simulink model "SerialComm"  (R2022a)
settings: Solver=FixedStepAuto  StartTime=0.0  StopTime=10.0  FixedStep=1e-3  RelTol=1e-3  EnableMultiTasking=on
undefined symbols (not defined in the file): A0, A1, D0, D1, D10, D11, D12, D13, D2, D3, D4, D5, D6, D7, D8, D9, PTA0, PTA1, PTA2, PTB2, PTB23, PTB3, PTB9, PTC16, PTC17, PTC2, PTC3, PTC4, PTD0, PTD1, PTD2, PTD3
libraries: frdmk64flib x19, svdutilitieslib x4, dspstat3 x1
settings Model: ExtModeTrigDuration=5  Creator=haotianxue  LastModifiedBy=1wanj
settings OptimizationCC: EnhancedBackFolding=on  PassReuseOutputArgsAs=Individual arguments  ZeroExternalMemoryAtStartup=off  ZeroInternalMemoryAtStartup=off  MaxStackSize=64  OptimizeBlockOrder=speed  DifferentSizesBufferReuse=on  OptimizationCustomize=off  EfficientTunableParamExpr=on
settings DebuggingCC: ParameterTunabilityLossMsg=error  UnconnectedInputMsg=warning  UnconnectedOutputMsg=warning  UnconnectedLineMsg=warning
settings HardwareCC: ProdBitPerPointer=32  ProdBitPerSizeT=32  ProdBitPerPtrDiffT=32  ProdLargestAtomicInteger=Long  ProdLargestAtomicFloat=Double  ProdWordSize=32  ProdHWDeviceType=ARM Compatible->ARM Cortex
settings SFSimCC: MATLABDynamicMemAlloc=off
settings RTWCC: SystemTargetFile=ert.tlc  HardwareBoard=NXP FRDM-K64F  TLCOptions="-aInlineSetEventsForThisBaseRateFcn=TLC_FALSE -aSuppressMultiTaskScheduler=TLC_FALSE  -aRateBasedStepFcn=0"  TemplateMakefile=ert_default_tmf  Toolchain=GNU Tools for ARM Embedded Processors  DLArmComputeVersion=19.05
settings CodeAppCC: ForceParamTrailComments=on  IgnoreCustomStorageClasses=off  OperatorAnnotations=on  SimulinkDataObjDesc=on  SFDataObjDesc=on  InsertBlockDesc=on
settings ERTTargetCC: ExtModeTransport=4  ExtModeMexFile=sendToCommService

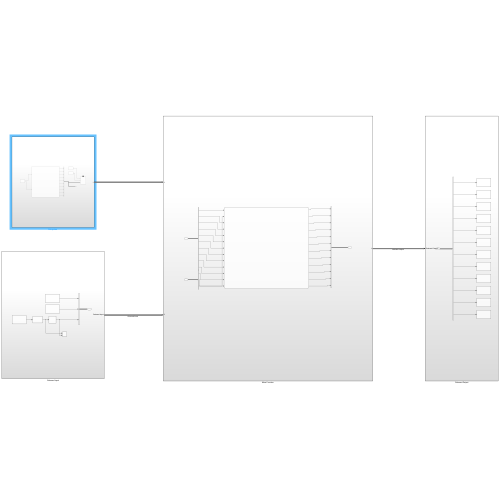
[thumbnail: Simulink's stored preview of the top-level diagram]
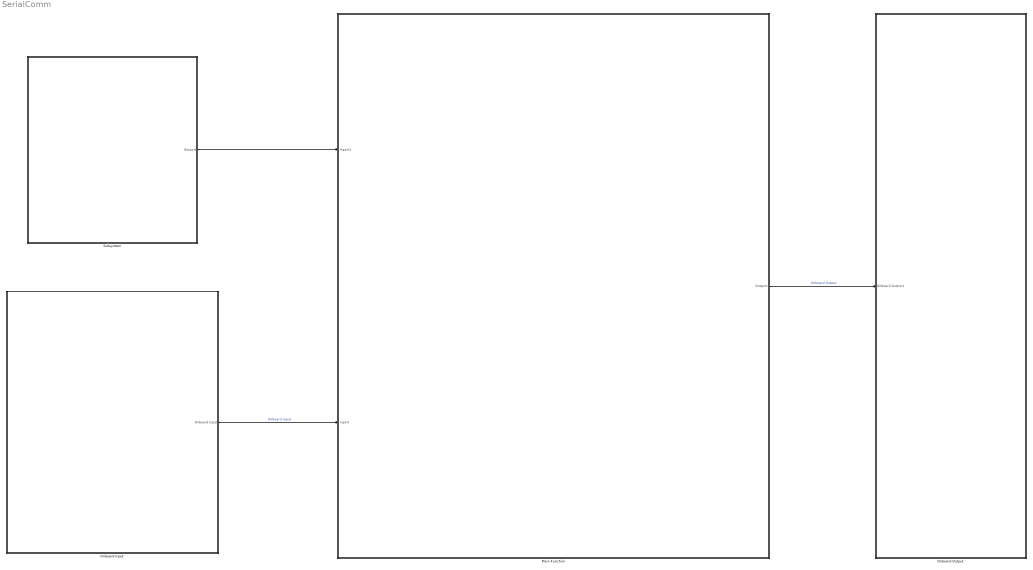
== system SerialComm ==
  Main Function : Subsystem
  Onboard Input : Subsystem
  Onboard Output : Subsystem
  Subsystem : Subsystem
  wires:
  Onboard Input/1(Onboard Input) -> Main Function/2(Inport)  "Onboard Input"
  Main Function/1(Outport) -> Onboard Output/1(Onboard Outport)  "Onboard Output"
  Subsystem/1(Outport) -> Main Function/1(Inport1)

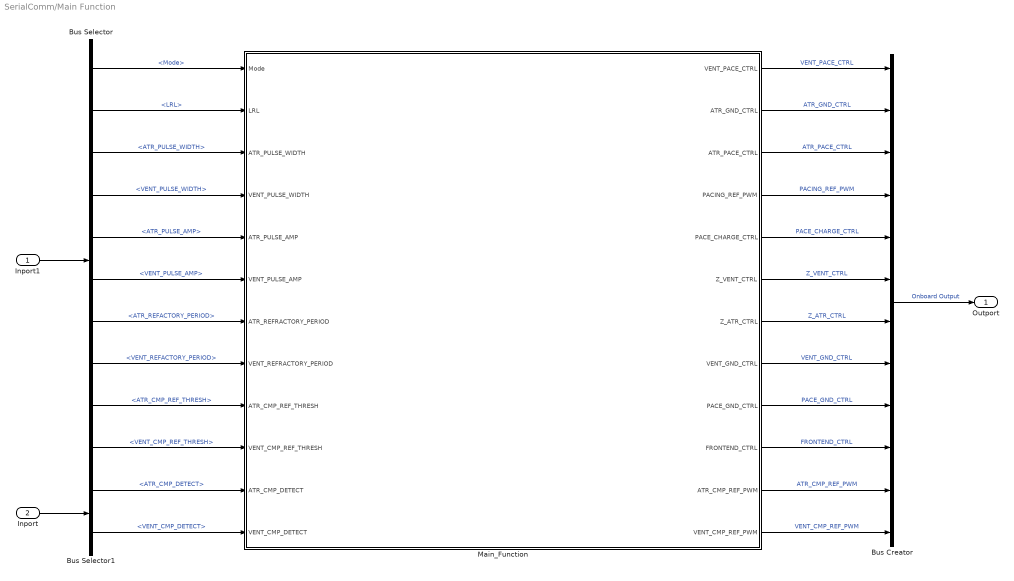
== system SerialComm/Main Function ==
  Inport1 : Inport
  Inport : Inport  Port=2
  Bus Creator : BusCreator  Inputs=12
  Bus Selector : BusSelector  OutputSignals=Mode,LRL,ATR_PULSE_WIDTH,VENT_PULSE_WIDTH,ATR_PULSE_AMP,VENT_PULSE_AMP,ATR_REFACTORY_PERIOD,VENT_REFACTORY_PERIOD,ATR_CMP_REF_THRESH,VENT_CMP_REF_THRESH
  Bus Selector1 : BusSelector  OutputSignals=ATR_CMP_DETECT,VENT_CMP_DETECT
  Main_Function : Stateflow chart  TreatAsAtomicUnit=on
  Outport : Outport
  wires:
  Main_Function/8(VENT_GND_CTRL) -> Bus Creator/8  "VENT_GND_CTRL"
  Main_Function/1(VENT_PACE_CTRL) -> Bus Creator/1  "VENT_PACE_CTRL"
  Bus Selector/1 -> Main_Function/1(Mode)  "<Mode>"
  Bus Selector/3 -> Main_Function/3(ATR_PULSE_WIDTH)  "<ATR_PULSE_WIDTH>"
  Bus Selector/4 -> Main_Function/4(VENT_PULSE_WIDTH)  "<VENT_PULSE_WIDTH>"
  Bus Selector1/1 -> Main_Function/11(ATR_CMP_DETECT)  "<ATR_CMP_DETECT>"
  Main_Function/9(PACE_GND_CTRL) -> Bus Creator/9  "PACE_GND_CTRL"
  Main_Function/7(Z_ATR_CTRL) -> Bus Creator/7  "Z_ATR_CTRL"
  Main_Function/6(Z_VENT_CTRL) -> Bus Creator/6  "Z_VENT_CTRL"
  Main_Function/5(PACE_CHARGE_CTRL) -> Bus Creator/5  "PACE_CHARGE_CTRL"
  Main_Function/4(PACING_REF_PWM) -> Bus Creator/4  "PACING_REF_PWM"
  Main_Function/3(ATR_PACE_CTRL) -> Bus Creator/3  "ATR_PACE_CTRL"
  Main_Function/2(ATR_GND_CTRL) -> Bus Creator/2  "ATR_GND_CTRL"
  Inport1/1 -> Bus Selector/1
  Inport/1 -> Bus Selector1/1
  Bus Creator/1 -> Outport/1  "Onboard Output"
  Bus Selector/5 -> Main_Function/5(ATR_PULSE_AMP)  "<ATR_PULSE_AMP>"
  Bus Selector/6 -> Main_Function/6(VENT_PULSE_AMP)  "<VENT_PULSE_AMP>"
  Main_Function/10(FRONTEND_CTRL) -> Bus Creator/10  "FRONTEND_CTRL"
  Main_Function/11(ATR_CMP_REF_PWM) -> Bus Creator/11  "ATR_CMP_REF_PWM"
  Main_Function/12(VENT_CMP_REF_PWM) -> Bus Creator/12  "VENT_CMP_REF_PWM"
  Bus Selector/9 -> Main_Function/9(ATR_CMP_REF_THRESH)  "<ATR_CMP_REF_THRESH>"
  Bus Selector/10 -> Main_Function/10(VENT_CMP_REF_THRESH)  "<VENT_CMP_REF_THRESH>"
  Bus Selector/2 -> Main_Function/2(LRL)  "<LRL>"
  Bus Selector1/2 -> Main_Function/12(VENT_CMP_DETECT)  "<VENT_CMP_DETECT>"
  Bus Selector/7 -> Main_Function/7(ATR_REFRACTORY_PERIOD)  "<ATR_REFACTORY_PERIOD>"
  Bus Selector/8 -> Main_Function/8(VENT_REFRACTORY_PERIOD)  "<VENT_REFACTORY_PERIOD>"

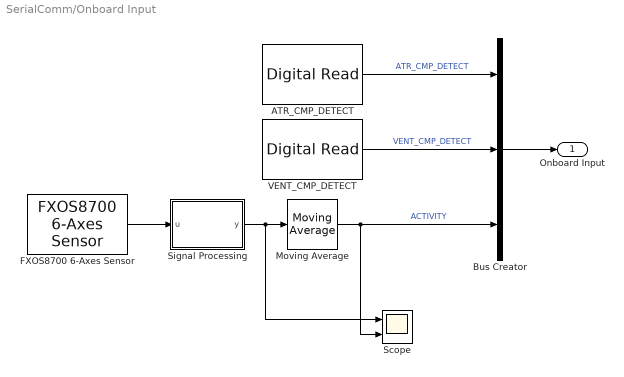
== system SerialComm/Onboard Input ==
  ATR_CMP_DETECT : frdmk64flib/Digital Read  Whichpin=PTC16 (D0)  SampleTime=-1
  Bus Creator : BusCreator  Inputs=3
  FXOS8700 6-Axes Sensor : frdmk64flib/FXOS8700 6-Axes Sensor  Activesensor=Accelerometer only  ODR=800Hz  HybridODR=400Hz  Accelfullrange=-4g to +4g  SampleTime=-1
  Moving Average : dspstat3/Moving Average  Method=Sliding window  ForgettingFactorPort=off  SpecifyWindowLength=on  WindowLength=30  ForgettingFactor=0.9  SimulateUsing=Code generation
  Scope : Scope  NumInputPorts=2
  Signal Processing : MATLAB Function  TreatAsAtomicUnit=on
  VENT_CMP_DETECT : frdmk64flib/Digital Read  Whichpin=PTC17 (D1)  SampleTime=-1
  Onboard Input : Outport
  wires:
  VENT_CMP_DETECT/1 -> Bus Creator/2  "VENT_CMP_DETECT"
  ATR_CMP_DETECT/1 -> Bus Creator/1  "ATR_CMP_DETECT"
  Bus Creator/1 -> Onboard Input/1
  FXOS8700 6-Axes Sensor/1 -> Signal Processing/1(u)
  Signal Processing/1(y) -> Scope/1, Moving Average/1
  Moving Average/1 -> Scope/2, Bus Creator/3  "ACTIVITY"

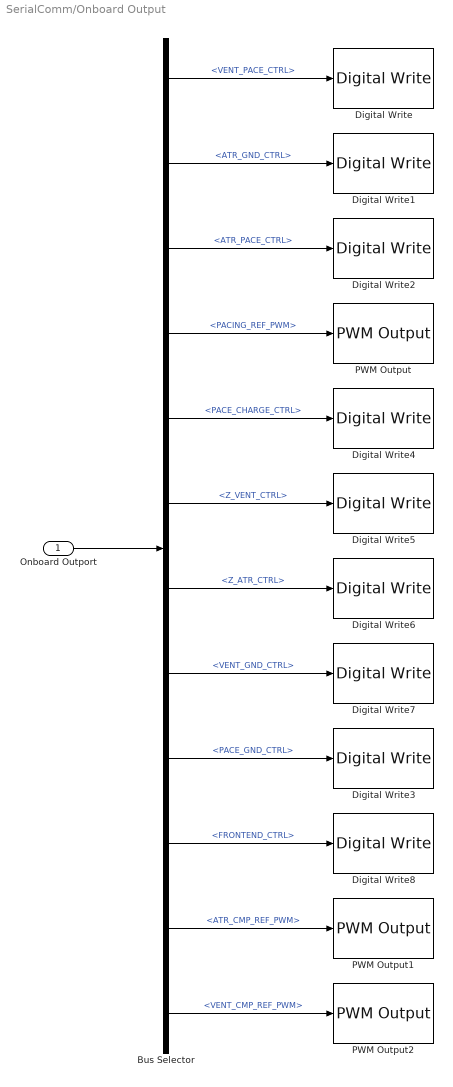
== system SerialComm/Onboard Output ==
  Onboard Outport : Inport
  Bus Selector : BusSelector  OutputSignals=VENT_PACE_CTRL,ATR_GND_CTRL,ATR_PACE_CTRL,PACING_REF_PWM,PACE_CHARGE_CTRL,Z_VENT_CTRL,Z_ATR_CTRL,VENT_GND_CTRL,PACE_GND_CTRL,FRONTEND_CTRL,ATR_CMP_REF_PWM,VENT_CMP_REF_PWM
  Digital Write : frdmk64flib/Digital Write  Whichpin=PTC4 (D9)
  Digital Write1 : frdmk64flib/Digital Write  Whichpin=PTD2 (D11)
  Digital Write2 : frdmk64flib/Digital Write  Whichpin=PTA0 (D8)
  Digital Write3 : frdmk64flib/Digital Write  Whichpin=PTD0 (D10)
  Digital Write4 : frdmk64flib/Digital Write  Whichpin=PTB9 (D2)
  Digital Write5 : frdmk64flib/Digital Write  Whichpin=PTC3 (D7)
  Digital Write6 : frdmk64flib/Digital Write  Whichpin=PTB23 (D4)
  Digital Write7 : frdmk64flib/Digital Write  Whichpin=PTD3 (D12)
  Digital Write8 : frdmk64flib/Digital Write  Whichpin=PTD1 (D13)
  PWM Output : frdmk64flib/PWM Output  Whichpin=PTA2 (D5)  InitialFrequency=2000  InitialDutyCycle=50
  PWM Output1 : frdmk64flib/PWM Output  Whichpin=PTC2 (D6)  InitialFrequency=2000  InitialDutyCycle=50
  PWM Output2 : frdmk64flib/PWM Output  Whichpin=PTA1 (D3)  InitialFrequency=2000  InitialDutyCycle=50
  wires:
  Onboard Outport/1 -> Bus Selector/1
  Bus Selector/1 -> Digital Write/1  "<VENT_PACE_CTRL>"
  Bus Selector/2 -> Digital Write1/1  "<ATR_GND_CTRL>"
  Bus Selector/3 -> Digital Write2/1  "<ATR_PACE_CTRL>"
  Bus Selector/4 -> PWM Output/1  "<PACING_REF_PWM>"
  Bus Selector/5 -> Digital Write4/1  "<PACE_CHARGE_CTRL>"
  Bus Selector/6 -> Digital Write5/1  "<Z_VENT_CTRL>"
  Bus Selector/7 -> Digital Write6/1  "<Z_ATR_CTRL>"
  Bus Selector/8 -> Digital Write7/1  "<VENT_GND_CTRL>"
  Bus Selector/9 -> Digital Write3/1  "<PACE_GND_CTRL>"
  Bus Selector/10 -> Digital Write8/1  "<FRONTEND_CTRL>"
  Bus Selector/11 -> PWM Output1/1  "<ATR_CMP_REF_PWM>"
  Bus Selector/12 -> PWM Output2/1  "<VENT_CMP_REF_PWM>"

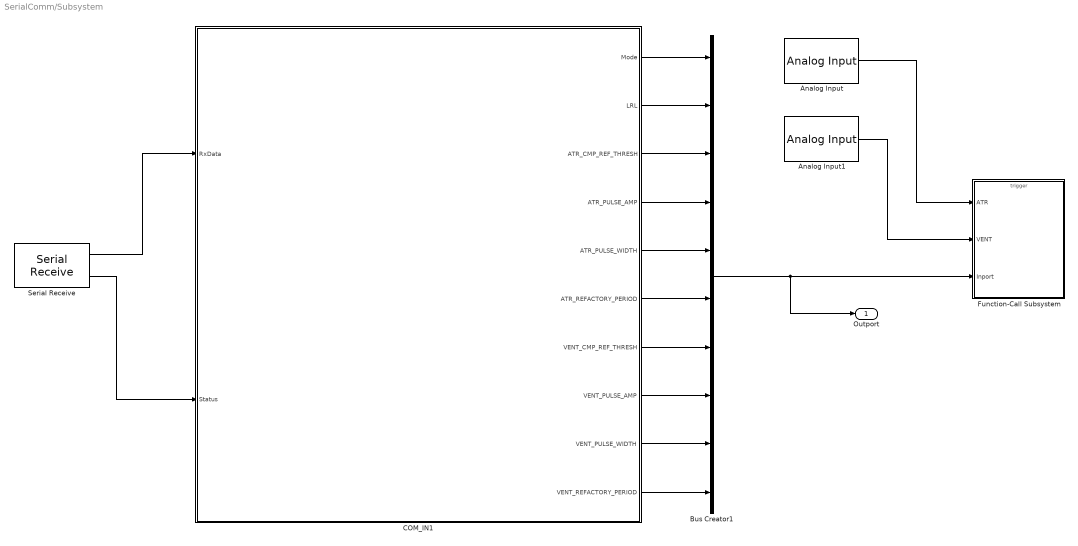
== system SerialComm/Subsystem ==
  Analog Input : frdmk64flib/Analog Input  Whichpin=PTB2 (A0)  SampleTime=-1
  Analog Input1 : frdmk64flib/Analog Input  Whichpin=PTB3 (A1)  SampleTime=-1
  Bus Creator1 : BusCreator  Inputs=10
  COM_IN1 : Stateflow chart  TreatAsAtomicUnit=on
  Function-Call Subsystem : Subsystem  TreatAsAtomicUnit=on
  Serial Receive : frdmk64flib/Serial Receive  SCIModule=0  Baudrate=uint32(9600)  Parity=None  StopBits=1  HardwareFlowControl=None  ByteOrder=LittleEndian  DataType=uint8  DataLength=14  BlockingMode=off  OutputStatus=on  SampleTime=-1
  Outport : Outport
  wires:
  Serial Receive/1 -> COM_IN1/1(RxData)
  Serial Receive/2 -> COM_IN1/2(Status)
  COM_IN1/1(Mode) -> Bus Creator1/1
  COM_IN1/2(LRL) -> Bus Creator1/2
  COM_IN1/3(ATR_CMP_REF_THRESH) -> Bus Creator1/3
  COM_IN1/4(ATR_PULSE_AMP) -> Bus Creator1/4
  COM_IN1/5(ATR_PULSE_WIDTH) -> Bus Creator1/5
  COM_IN1/6(ATR_REFACTORY_PERIOD) -> Bus Creator1/6
  COM_IN1/7(VENT_CMP_REF_THRESH) -> Bus Creator1/7
  COM_IN1/8(VENT_PULSE_AMP) -> Bus Creator1/8
  COM_IN1/9(VENT_PULSE_WIDTH) -> Bus Creator1/9
  COM_IN1/10(VENT_REFACTORY_PERIOD) -> Bus Creator1/10
  Bus Creator1/1 -> Outport/1, Function-Call Subsystem/3(Inport)
  Analog Input/1 -> Function-Call Subsystem/1(ATR)
  Analog Input1/1 -> Function-Call Subsystem/2(VENT)

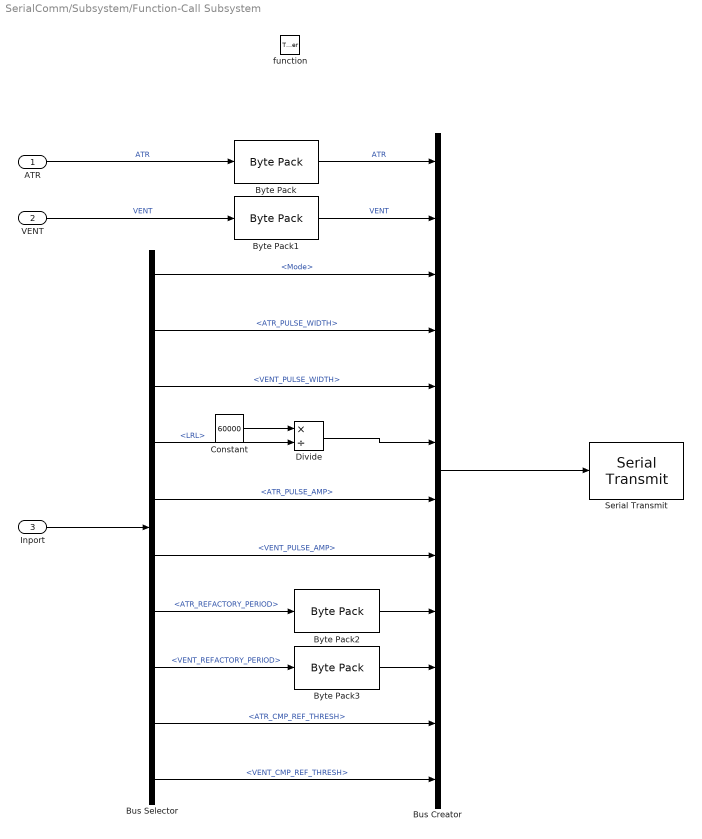
== system SerialComm/Subsystem/Function-Call Subsystem ==
  ATR : Inport  OutDataTypeStr=double
  VENT : Inport  Port=2  OutDataTypeStr=double
  Inport : Inport  Port=3
  function : TriggerPort  TriggerType=function-call  IsSimulinkFunction=on  FunctionName=Send_Data  VariantControl=(inherit)
  Bus Creator : BusCreator  Inputs=12
  Bus Selector : BusSelector  OutputSignals=Mode,ATR_PULSE_WIDTH,VENT_PULSE_WIDTH,LRL,ATR_PULSE_AMP,VENT_PULSE_AMP,ATR_REFACTORY_PERIOD,VENT_REFACTORY_PERIOD,ATR_CMP_REF_THRESH,VENT_CMP_REF_THRESH
  Byte Pack : svdutilitieslib/Byte Pack  maskPackedDataType=uint8  datatypes={'double'}  byteAlign=1  blockPlatform=arduinoert
      settings: SourceProductBaseCode=ANDROID,ARDUINO,ML_ARDUINO,ECCORTEXA,ECCORTEXR,SC_BEAGLEBONE_BLUE,EC_FREEDOM_BOARD,EC_FRDM_K64F,INTEL_BLOCKSET,MICROBIT,NUCLEO,NVIDIA,PX4AUTOPILOTS,RASPPIIO,STMICRODIS,TIC2000,XILINX_BLOCKSET
  Byte Pack1 : svdutilitieslib/Byte Pack  maskPackedDataType=uint8  datatypes={'double'}  byteAlign=1  blockPlatform=arduinoert
      settings: SourceProductBaseCode=ANDROID,ARDUINO,ML_ARDUINO,ECCORTEXA,ECCORTEXR,SC_BEAGLEBONE_BLUE,EC_FREEDOM_BOARD,EC_FRDM_K64F,INTEL_BLOCKSET,MICROBIT,NUCLEO,NVIDIA,PX4AUTOPILOTS,RASPPIIO,STMICRODIS,TIC2000,XILINX_BLOCKSET
  Byte Pack2 : svdutilitieslib/Byte Pack  maskPackedDataType=uint8  datatypes={'uint16'}  byteAlign=1  blockPlatform=arduinoert
      settings: SourceProductBaseCode=ANDROID,ARDUINO,ML_ARDUINO,ECCORTEXA,ECCORTEXR,SC_BEAGLEBONE_BLUE,EC_FREEDOM_BOARD,EC_FRDM_K64F,INTEL_BLOCKSET,MICROBIT,NUCLEO,NVIDIA,PX4AUTOPILOTS,RASPPIIO,STMICRODIS,TIC2000,XILINX_BLOCKSET
  Byte Pack3 : svdutilitieslib/Byte Pack  maskPackedDataType=uint8  datatypes={'uint16'}  byteAlign=1  blockPlatform=arduinoert
      settings: SourceProductBaseCode=ANDROID,ARDUINO,ML_ARDUINO,ECCORTEXA,ECCORTEXR,SC_BEAGLEBONE_BLUE,EC_FREEDOM_BOARD,EC_FRDM_K64F,INTEL_BLOCKSET,MICROBIT,NUCLEO,NVIDIA,PX4AUTOPILOTS,RASPPIIO,STMICRODIS,TIC2000,XILINX_BLOCKSET
  Constant : Constant  Value=60000
  Divide : Product  Inputs=*/  OutDataTypeStr=uint8
  Serial Transmit : frdmk64flib/Serial Transmit  SCIModule=0  Baudrate=uint32(9600)  Parity=None  StopBits=1  HardwareFlowControl=None  ByteOrder=LittleEndian  BlockingMode=on  OutputStatus=off
  wires:
  Inport/1 -> Bus Selector/1
  Bus Selector/1 -> Bus Creator/3  "<Mode>"
  Byte Pack/1 -> Bus Creator/1  "ATR"
  ATR/1 -> Byte Pack/1  "ATR"
  Byte Pack1/1 -> Bus Creator/2  "VENT"
  Bus Creator/1 -> Serial Transmit/1
  VENT/1 -> Byte Pack1/1  "VENT"
  Bus Selector/2 -> Bus Creator/4  "<ATR_PULSE_WIDTH>"
  Bus Selector/3 -> Bus Creator/5  "<VENT_PULSE_WIDTH>"
  Bus Selector/7 -> Byte Pack2/1  "<ATR_REFACTORY_PERIOD>"
  Bus Selector/5 -> Bus Creator/7  "<ATR_PULSE_AMP>"
  Bus Selector/6 -> Bus Creator/8  "<VENT_PULSE_AMP>"
  Bus Selector/8 -> Byte Pack3/1  "<VENT_REFACTORY_PERIOD>"
  Bus Selector/9 -> Bus Creator/11  "<ATR_CMP_REF_THRESH>"
  Bus Selector/10 -> Bus Creator/12  "<VENT_CMP_REF_THRESH>"
  Byte Pack2/1 -> Bus Creator/9
  Byte Pack3/1 -> Bus Creator/10
  Bus Selector/4 -> Divide/2  "<LRL>"
  Divide/1 -> Bus Creator/6
  Constant/1 -> Divide/1

== stateflow chart SerialComm/Main Function/Main_Function ==
  state AAI_Mode
    entry:
    ATR_PACE_CTRL = 0;
    ATR_GND_CTRL = 1;
    %
    VENT_PACE_CTRL = 0;
    VENT_GND_CTRL = 0;
    %
    PACING_REF_PWM = ATR_PULSE_AMP;
    ATR_CMP_REF_PWM = ATR_CMP_REF_THRESH;
    PACE_CHARGE_CTRL = 1;
    %
    Z_VENT_CTRL = 0;
    Z_ATR_CTRL = 0;
    %
    FRONTEND_CTRL = 1; %was 0
    state SendPulse
      entry:
      PACE_CHARGE_CTRL = 0;
      PACE_GND_CTRL = 1;
      ATR_PACE_CTRL = 1;
      ATR_GND_CTRL = 0;
      VENT_PACE_CTRL = 0;
      VENT_GND_CTRL = 0;
      FRONTEND_CTRL = 1; %was 0
    state ReadyPulse
      entry:
      PACE_CHARGE_CTRL = 1;
      PACE_GND_CTRL = 1;
      ATR_PACE_CTRL = 0;
      ATR_GND_CTRL = 1;
      VENT_PACE_CTRL = 0;
      VENT_GND_CTRL = 0;
      FRONTEND_CTRL = 1;
    (default) -> AAI_Mode.ReadyPulse
    AAI_Mode.SendPulse -> AAI_Mode.ReadyPulse : after(ATR_PULSE_WIDTH,msec)
    AAI_Mode.ReadyPulse -> AAI_Mode.SendPulse [order 2] : after(LRL-ATR_REFRACTORY_PERIOD-uint16(ATR_PULSE_WIDTH),msec)
    AAI_Mode.ReadyPulse -> AAI_Mode.ReadyPulse [order 1] : after(ATR_REFRACTORY_PERIOD,msec)[ATR_CMP_DETECT == true]
  state AOO_Mode
    entry:
    ATR_PACE_CTRL = 0;
    ATR_GND_CTRL = 1;
    %
    VENT_PACE_CTRL = 0;
    VENT_GND_CTRL = 0;
    %
    PACING_REF_PWM = ATR_PULSE_AMP;
    PACE_CHARGE_CTRL = 1;
    %
    Z_VENT_CTRL = 0;
    Z_ATR_CTRL = 0;
    state ReadyPulse
      entry:
      PACE_CHARGE_CTRL = 1;
      PACE_GND_CTRL = 1;
      ATR_PACE_CTRL = 0;
      ATR_GND_CTRL = 1;
      VENT_PACE_CTRL = 0;
      VENT_GND_CTRL = 0;
    state SendPulse
      entry:
      PACE_CHARGE_CTRL = 0;
      PACE_GND_CTRL = 1;
      ATR_PACE_CTRL = 1;
      ATR_GND_CTRL = 0;
      VENT_PACE_CTRL = 0;
      VENT_GND_CTRL = 0;
    (default) -> AOO_Mode.ReadyPulse
    AOO_Mode.ReadyPulse -> AOO_Mode.SendPulse : after(LRL - uint16(ATR_PULSE_WIDTH),msec)
    AOO_Mode.SendPulse -> AOO_Mode.ReadyPulse : after(ATR_PULSE_WIDTH,msec)
  state AAI_Mode1 [commented out]
    entry:
    ATR_CMP_REF_PWM = ATR_CMP_REF_THRESH*20;
    %
    PACING_REF_PWM = ATR_PULSE_AMP*20;
    PACE_GND_CTRL = 1;
    Z_VENT_CTRL = 0;
    Z_ATR_CTRL = 0;
    %
    FRONTEND_CTRL = 1;
    state Pace [commented out]
      entry:
      PACE_CHARGE_CTRL = 0;
      ATR_PACE_CTRL = 1;
      ATR_GND_CTRL = 0;
    state Charge [commented out]
      entry:
      PACE_CHARGE_CTRL = 1;
      ATR_PACE_CTRL = 0;
      ATR_GND_CTRL = 1;
    AAI_Mode1.Pace -> AAI_Mode1.Charge [commented out] : after(ATR_PULSE_WIDTH,msec)
    (default) -> AAI_Mode1.Charge [commented out]
    AAI_Mode1.Charge -> AAI_Mode1.Charge [commented out] : after(ATR_REFRACTORY_PERIOD,msec)[ATR_CMP_DETECT == true]
    AAI_Mode1.Charge -> AAI_Mode1.Pace [commented out] : after(60*1000/PACING_RATE-ATR_REFRACTORY_PERIOD-uint16(ATR_PULSE_WIDTH),msec)
  state AOO_Mode1 [commented out]
    entry:
    PACING_REF_PWM = ATR_PULSE_AMP*20;
    PACE_GND_CTRL = 1;
    %
    Z_VENT_CTRL = 0;
    Z_ATR_CTRL = 0;
    state Charge [commented out]
      entry:
      PACE_CHARGE_CTRL = 1;
      ATR_PACE_CTRL = 0;
      ATR_GND_CTRL = 1;
    state Pace [commented out]
      entry:
      PACE_CHARGE_CTRL = 0;
      ATR_PACE_CTRL = 1;
      ATR_GND_CTRL = 0;
    (default) -> AOO_Mode1.Charge [commented out]
    AOO_Mode1.Pace -> AOO_Mode1.Charge [commented out] : after(ATR_PULSE_WIDTH,msec)
    AOO_Mode1.Charge -> AOO_Mode1.Pace [commented out] : after(60*1000/PACING_RATE - uint16(ATR_PULSE_WIDTH),msec)
  state Mode_Selector
    entry:
    ATR_PACE_CTRL = 0;
    ATR_GND_CTRL = 0;
    %
    VENT_PACE_CTRL = 0;
    VENT_GND_CTRL = 0;
    %
    PACE_CHARGE_CTRL = 0;
    PACE_GND_CTRL = 0;
    %
    Z_VENT_CTRL = 0;
    Z_ATR_CTRL = 0;
    %
    FRONTEND_CTRL = 1; %was 0
  state OFF [commented out]
    entry:
    PACE_CHARGE_CTRL = 0;
    PACE_GND_CTRL = 0;
    Z_VENT_CTRL = 0;
    Z_ATR_CTRL = 0;
    %
    FRONTEND_CTRL = 0;
    %
    ATR_PACE_CTRL = 0;
    ATR_GND_CTRL = 0;
    VENT_PACE_CTRL = 0;
    VENT_GND_CTRL = 0;
    %
    PACING_RATE = uint16(LRL);
  state VVI_Mode
    entry:
    VENT_PACE_CTRL = 0;
    VENT_GND_CTRL = 1;
    %
    ATR_PACE_CTRL = 0;
    ATR_GND_CTRL = 0;
    %
    PACING_REF_PWM = VENT_PULSE_AMP;
    VENT_CMP_REF_PWM = VENT_CMP_REF_THRESH;
    PACE_CHARGE_CTRL = 1;
    %
    Z_VENT_CTRL = 0;
    Z_ATR_CTRL = 0;
    %
    FRONTEND_CTRL = 1;
    state SendPulse
      entry:
      PACE_CHARGE_CTRL = 0;
      PACE_GND_CTRL = 1;
      VENT_PACE_CTRL = 1;
      VENT_GND_CTRL = 0;
      ATR_PACE_CTRL = 0;
      ATR_GND_CTRL = 0;
      FRONTEND_CTRL = 1; %was 0
    state ReadyPulse
      entry:
      PACE_CHARGE_CTRL = 1;
      PACE_GND_CTRL = 1;
      VENT_PACE_CTRL = 0;
      VENT_GND_CTRL = 1;
      ATR_PACE_CTRL = 0;
      ATR_GND_CTRL = 0;
      FRONTEND_CTRL = 1;
    (default) -> VVI_Mode.ReadyPulse
    VVI_Mode.SendPulse -> VVI_Mode.ReadyPulse : after(VENT_PULSE_WIDTH,msec)
    VVI_Mode.ReadyPulse -> VVI_Mode.SendPulse [order 2] : after(LRL - VENT_REFRACTORY_PERIOD - uint16(VENT_PULSE_WIDTH),msec)
    VVI_Mode.ReadyPulse -> VVI_Mode.ReadyPulse [order 1] : after(VENT_REFRACTORY_PERIOD,msec)[VENT_CMP_DETECT == true]
  state VOO_Mode
    entry:
    ATR_PACE_CTRL = 0;
    ATR_GND_CTRL = 0;
    %
    VENT_PACE_CTRL = 0;
    VENT_GND_CTRL = 1;
    %
    PACING_REF_PWM = VENT_PULSE_AMP;
    PACE_CHARGE_CTRL = 1;
    %
    Z_VENT_CTRL = 0;
    Z_ATR_CTRL = 0;
    state ReadyPulse
      entry:
      PACE_CHARGE_CTRL = 1;
      PACE_GND_CTRL = 1;
      ATR_PACE_CTRL = 0;
      ATR_GND_CTRL = 0;
      VENT_PACE_CTRL = 0;
      VENT_GND_CTRL = 1;
    state SendPulse
      entry:
      PACE_CHARGE_CTRL = 0;
      PACE_GND_CTRL = 1;
      ATR_PACE_CTRL = 0;
      ATR_GND_CTRL = 0;
      VENT_PACE_CTRL = 1;
      VENT_GND_CTRL = 0;
    (default) -> VOO_Mode.ReadyPulse
    VOO_Mode.SendPulse -> VOO_Mode.ReadyPulse : after(VENT_PULSE_WIDTH,msec)
    VOO_Mode.ReadyPulse -> VOO_Mode.SendPulse : after(LRL - uint16(VENT_PULSE_WIDTH),msec)
  state VVI_Mode1 [commented out]
    entry:
    VENT_CMP_REF_PWM = VENT_CMP_REF_THRESH*20;
    %
    PACING_REF_PWM = VENT_PULSE_AMP*20;
    PACE_GND_CTRL = 1;
    Z_VENT_CTRL = 0;
    Z_ATR_CTRL = 0;
    %
    FRONTEND_CTRL = 1;
    state Charge [commented out]
      entry:
      PACE_CHARGE_CTRL = 1;
      VENT_PACE_CTRL = 0;
      VENT_GND_CTRL = 1;
    state Pace [commented out]
      entry:
      PACE_CHARGE_CTRL = 0;
      VENT_PACE_CTRL = 1;
      VENT_GND_CTRL = 0;
    VVI_Mode1.Pace -> VVI_Mode1.Charge [commented out] : after(VENT_PULSE_WIDTH,msec)
    (default) -> VVI_Mode1.Charge [commented out]
    VVI_Mode1.Charge -> VVI_Mode1.Pace [commented out] : after(60*1000/PACING_RATE-VENT_REFRACTORY_PERIOD-uint16(VENT_PULSE_WIDTH),msec)
    VVI_Mode1.Charge -> VVI_Mode1.Charge [commented out] : after(VENT_REFRACTORY_PERIOD,msec)[VENT_CMP_DETECT == true]
  state VOO_Mode1 [commented out]
    entry:
    PACING_REF_PWM = VENT_PULSE_AMP*20;
    PACE_GND_CTRL = 1;
    %
    Z_VENT_CTRL = 0;
    Z_ATR_CTRL = 0;
    state Charge [commented out]
      entry:
      PACE_CHARGE_CTRL = 1;
      VENT_PACE_CTRL = 0;
      VENT_GND_CTRL = 1;
    state Pace [commented out]
      entry:
      PACE_CHARGE_CTRL = 0;
      VENT_PACE_CTRL = 1;
      VENT_GND_CTRL = 0;
    (default) -> VOO_Mode1.Charge [commented out]
    VOO_Mode1.Pace -> VOO_Mode1.Charge [commented out] : after(VENT_PULSE_WIDTH,msec)
    VOO_Mode1.Charge -> VOO_Mode1.Pace [commented out] : after(60*1000/PACING_RATE - uint16(VENT_PULSE_WIDTH),msec)
  Mode_Selector -> AAI_Mode [order 4] : [Mode == 3]
  Mode_Selector -> AOO_Mode [order 1] : [Mode == 1]
  AAI_Mode -> Mode_Selector : [Mode ~= 3]
  (default) -> Mode_Selector
  AOO_Mode -> Mode_Selector : [Mode ~= 1]
  (default) -> OFF [commented out]
  OFF -> AOO_Mode1 [commented out] : [Mode == 1]
  OFF -> AAI_Mode1 [commented out] : [Mode == 3]
  VVI_Mode -> Mode_Selector : [Mode ~= 4]
  AOO_Mode1 -> OFF [commented out] : [Mode ~= 1]
  AAI_Mode1 -> OFF [commented out] : [Mode ~= 3]
  Mode_Selector -> VVI_Mode [order 3] : [Mode == 4]
  Mode_Selector -> VOO_Mode [order 2] : [Mode == 2]
  VOO_Mode -> Mode_Selector : [Mode ~= 2]
  VVI_Mode1 -> OFF [commented out] : [Mode == 4]
  VOO_Mode1 -> OFF [commented out] : [Mode == 2]
  OFF -> VOO_Mode1 [commented out] : [Mode ~= 2]
  OFF -> VVI_Mode1 [commented out] : [Mode ~= 4]
  data: VENT_PACE_CTRL output double; ATR_GND_CTRL output double; ATR_PACE_CTRL output double; PACING_REF_PWM output uint8; PACE_CHARGE_CTRL output double; Z_VENT_CTRL output double; Z_ATR_CTRL output double; VENT_GND_CTRL output double; Mode input uint8; LRL input uint16; PACE_GND_CTRL output double; ATR_PULSE_WIDTH input uint8 =0.4; VENT_PULSE_WIDTH input uint8 =0.4; ATR_PULSE_AMP input uint8; VENT_PULSE_AMP input uint8; ATR_REFRACTORY_PERIOD input; VENT_REFRACTORY_PERIOD input; ATR_CMP_REF_THRESH input uint8; VENT_CMP_REF_THRESH input uint8; ATR_CMP_DETECT input; VENT_CMP_DETECT input; FRONTEND_CTRL output double; ATR_CMP_REF_PWM output uint8; VENT_CMP_REF_PWM output uint8

== matlab function SerialComm/Onboard Input/Signal Processing ==
  data: u input; y output
function y = fcn(u)
y = 8*norm(u);

== stateflow chart SerialComm/Subsystem/COM_IN1 ==
  settings: executeAtInitialization=1
  state SET_VELUE
    entry:
    Mode = RxData(3);
    ATR_PULSE_WIDTH = RxData(4);
    VENT_PULSE_WIDTH = RxData(5);
    LRL = 60000/uint16(RxData(6));
    ATR_PULSE_AMP = RxData(7)*20 ;
    VENT_PULSE_AMP = RxData(8)*20;
    ATR_REFACTORY_PERIOD = typecast(RxData(9:10),'uint16');
    VENT_REFACTORY_PERIOD = typecast(RxData(11:12),'uint16');
    ATR_CMP_REF_THRESH = RxData(13)*20;
    VENT_CMP_REF_THRESH = RxData(14)*20;
  state INILIZATION
    entry:
    Mode = 3;
    ATR_PULSE_WIDTH = 1;
    VENT_PULSE_WIDTH = 1;
    LRL = 60000/60;
    ATR_PULSE_AMP = 60;
    VENT_PULSE_AMP = 60;
    ATR_REFACTORY_PERIOD = 250;
    VENT_REFACTORY_PERIOD =320;
    ATR_CMP_REF_THRESH = 80;
    VENT_CMP_REF_THRESH = 80;
  state STANDBY
    %Waiting for COM
  state SEND_VALUE
    entry: Send_Data();
  SET_VELUE -> STANDBY
  (junction 77) -> SET_VELUE [order 1] : [RxData(2) == 5]
  (default) -> INILIZATION
  (junction 77) -> STANDBY [order 3]
  INILIZATION -> STANDBY
  STANDBY -> (junction 77) : [Status == 0 && length(RxData) == 14 && RxData(1) == 12]
  (junction 77) -> SEND_VALUE [order 2] : [RxData(2) == 15]
  SEND_VALUE -> STANDBY
  data: RxData input uint8; Status input uint8; Mode output uint8; LRL output uint16; ATR_CMP_REF_THRESH output uint8; ATR_PULSE_AMP output uint8; ATR_PULSE_WIDTH output uint8; ATR_REFACTORY_PERIOD output uint16; VENT_CMP_REF_THRESH output uint8; VENT_PULSE_AMP output uint8; VENT_PULSE_WIDTH output uint8; VENT_REFACTORY_PERIOD output uint16
